simulink model "ModeStEnCtrl4s"  (R2018b)
settings: Solver=FixedStepDiscrete  StartTime=0.0  StopTime=10.0  FixedStep=0.01  RelTol=1e-3
undefined symbols (not defined in the file): EZE4sLStEnCtrl_Cal, EZE4sRStEnCtrl_Cal, EZQ4sLStEnCtrl_Cal, EZQ4sRStEnCtrl_Cal, FirstTrig, FwdLStEnCtrl_Cal, FwdRStEnCtrl_Cal, LgrstClsLStEnCtrl_Cal, LgrstClsRStEnCtrl_Cal, LgrstOpnLStEnCtrl_Cal, LgrstOpnRStEnCtrl_Cal, LyLStEnCtrl_Cal, LyRStEnCtrl_Cal, RecvL4sStEnCtrl_Cal, RecvR4sStEnCtrl_Cal, ResetCond, VIPL3582StEnCtrl_Cal, VIPL4sStEnCtrl_Cal, VIPR3582StEnCtrl_Cal, VIPR4sStEnCtrl_Cal, WelcomeBkwdStEnCtrl_Cal, WelcomeFwdStEnCtrl_Cal
libraries: simulink x20
settings Model: ModifiedHistory=2023.8.1 V2.0.0 CR421790 增加模式21-26  Creator=sn2xws  LastModifiedBy=sn55gm
settings DataIOCC: SaveFormat=StructureWithTime
settings OptimizationCC: DefaultParameterBehavior=Inlined  EnhancedBackFolding=on  PassReuseOutputArgsAs=Individual arguments  ZeroExternalMemoryAtStartup=off  ZeroInternalMemoryAtStartup=off  OptimizeBlockOrder=speed  DifferentSizesBufferReuse=on  OptimizationCustomize=off
settings DebuggingCC: ParameterTunabilityLossMsg=error
settings SFSimCC: MATLABDynamicMemAlloc=off
settings RTWCC: SystemTargetFile=autosar.tlc  GenCodeOnly=on  TemplateMakefile=ert_default_tmf  Description=AUTOSAR  GenerateReport=on  IncludeHyperlinkInReport=on  LaunchReport=on  GenerateTraceInfo=on  GenerateTraceReport=on  GenerateTraceReportSl=on  GenerateTraceReportSf=on  GenerateTraceReportEml=on  GenerateCodeMetricsReport=on
settings CodeAppCC: ForceParamTrailComments=on  IgnoreCustomStorageClasses=off  OperatorAnnotations=on  SimulinkDataObjDesc=on  SFDataObjDesc=on  InsertBlockDesc=on
settings STFCustomTargetCC: TargetLangStandard=C99 (ISO)  MultiwordLength=256  ParMdlRefBuildCompliant=on  CompOptLevelCompliant=on  IncludeMdlTerminateFcn=off  CombineOutputUpdateFcns=on  SuppressErrorStatus=on  ERTCustomFileBanners=on  SupportNonFinite=off  SupportComplex=off  SupportContinuousTime=off  SupportNonInlinedSFcns=off  RemoveResetFunc=on  MATLABClassNameForMDSCustomization=Simulink.SoftwareTarget.ERTCustomization  AutosarCompliant=on  UseToolchainInfoCompliant=on  LookupTableObjectStructAxisOrder=2,1,3,4,...  LUTObjectStructOrderEvenSpacing=Size,Table,Breakpoints  SystemTargetFile=autosar.tlc
settings ERTTargetCC: TargetLangStandard=C99 (ISO)  ConcurrentExecutionCompliant=off  IncludeMdlTerminateFcn=off  SuppressErrorStatus=on  SupportNonFinite=off  SupportComplex=off  ModelStepFunctionPrototypeControlCompliant=off  CPPClassGenCompliant=off  AutosarCompliant=on  LookupTableObjectStructAxisOrder=2,1,3,4,...  LUTObjectStructOrderEvenSpacing=Size,Table,Breakpoints  InlinedParameterPlacement=NonHierarchical  ERTCustomFileTemplate=example_file_process.tlc  ERTFilePackagingFormat=Compact

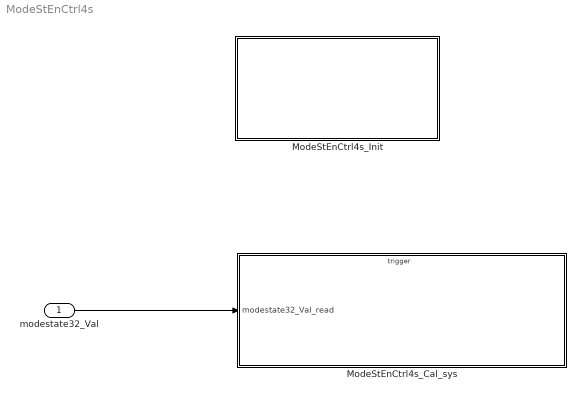
== system ModeStEnCtrl4s ==
  modestate32_Val : Inport  OutDataTypeStr=uint32  PortDimensions=1
  ModeStEnCtrl4s_Cal_sys : Subsystem
  ModeStEnCtrl4s_Init : Subsystem
  wires:
  modestate32_Val/1 -> ModeStEnCtrl4s_Cal_sys/1(modestate32_Val_read)

== system ModeStEnCtrl4s/ModeStEnCtrl4s_Cal_sys ==
  modestate32_Val_read : Inport
  function : TriggerPort  TriggerType=function-call  IsSimulinkFunction=on  FunctionName=ModeStEnCtrl4s_Cal  VariantControl=(inherit)
  Subsystem : Subsystem
  wires:
  modestate32_Val_read/1 -> Subsystem/1(modestate32_Val_read)

== system ModeStEnCtrl4s/ModeStEnCtrl4s_Init ==
  Event Listener : EventListener  EventName=reset

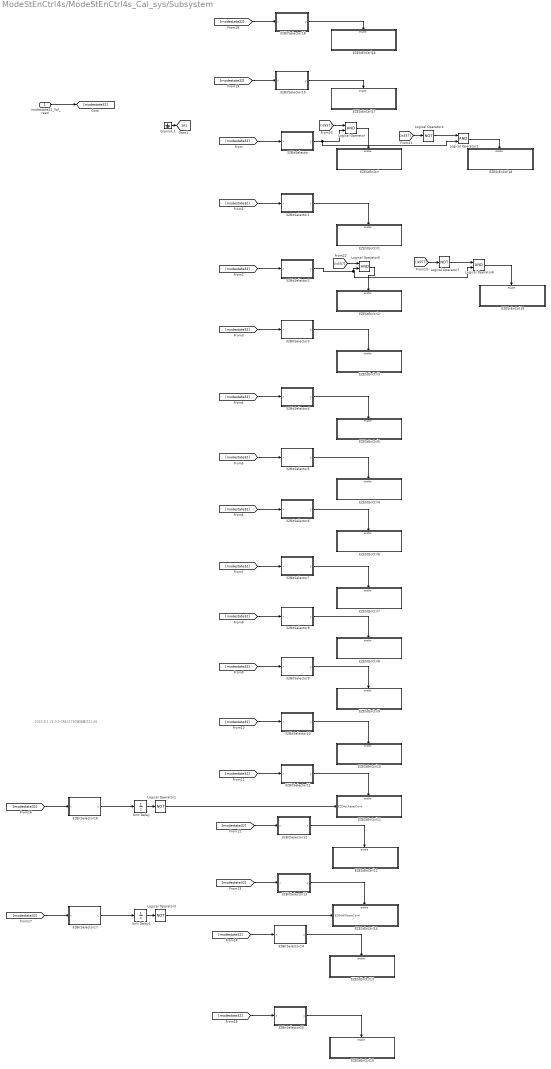
== system ModeStEnCtrl4s/ModeStEnCtrl4s_Cal_sys/Subsystem ==
  note: 2023.8.1 V2.0.0 CR421790 增加模式21-26
  modestate32_Val_read : Inport
  32BitSelector : Subsystem  mask(32 Bit Selector){BitNum=9}
      mask prompts: BitNum "Select Bit Number"
      mask help: Allows selection of a particular bit (0-31) out of a packed word up to 32 bits long. Output will be true if the bit number selected via the mask parameter is equal to one.
      mask TypeOptions BitNum: 0 | 1 | 2 | 3 | 4 | 5 | 6 | 7 | 8 | 9 | 10 | 11 | 12 | 13 | 14 | 15 | 16 | 17 | 18 | 19 | 20 | 21 | 22 | 23 | 24 | 25 | 26 | 27 | 28 | 29 | 30 | 31
      mask Display:
      | text(0.5, 0.8,'BIT','horizontalAlignment','center')
      | text(0.5, 0.5,'SELECTOR','horizontalAlignment','center')
      | text(0.5, 0.2,['-- Bit ',char(get_param(gcb,'BitNum')),' --'],'horizontalAlignment','center')
  32BitSelector1 : Subsystem  mask(32 Bit Selector){BitNum=10}
      mask prompts: BitNum "Select Bit Number"
      mask help: Allows selection of a particular bit (0-31) out of a packed word up to 32 bits long. Output will be true if the bit number selected via the mask parameter is equal to one.
      mask TypeOptions BitNum: 0 | 1 | 2 | 3 | 4 | 5 | 6 | 7 | 8 | 9 | 10 | 11 | 12 | 13 | 14 | 15 | 16 | 17 | 18 | 19 | 20 | 21 | 22 | 23 | 24 | 25 | 26 | 27 | 28 | 29 | 30 | 31
      mask Display:
      | text(0.5, 0.8,'BIT','horizontalAlignment','center')
      | text(0.5, 0.5,'SELECTOR','horizontalAlignment','center')
      | text(0.5, 0.2,['-- Bit ',char(get_param(gcb,'BitNum')),' --'],'horizontalAlignment','center')
  32BitSelector10 : Subsystem  mask(32 Bit Selector){BitNum=20}
      mask prompts: BitNum "Select Bit Number"
      mask help: Allows selection of a particular bit (0-31) out of a packed word up to 32 bits long. Output will be true if the bit number selected via the mask parameter is equal to one.
      mask TypeOptions BitNum: 0 | 1 | 2 | 3 | 4 | 5 | 6 | 7 | 8 | 9 | 10 | 11 | 12 | 13 | 14 | 15 | 16 | 17 | 18 | 19 | 20 | 21 | 22 | 23 | 24 | 25 | 26 | 27 | 28 | 29 | 30 | 31
      mask Display:
      | text(0.5, 0.8,'BIT','horizontalAlignment','center')
      | text(0.5, 0.5,'SELECTOR','horizontalAlignment','center')
      | text(0.5, 0.2,['-- Bit ',char(get_param(gcb,'BitNum')),' --'],'horizontalAlignment','center')
  32BitSelector11 : Subsystem  mask(32 Bit Selector){BitNum=21}
      mask prompts: BitNum "Select Bit Number"
      mask help: Allows selection of a particular bit (0-31) out of a packed word up to 32 bits long. Output will be true if the bit number selected via the mask parameter is equal to one.
      mask TypeOptions BitNum: 0 | 1 | 2 | 3 | 4 | 5 | 6 | 7 | 8 | 9 | 10 | 11 | 12 | 13 | 14 | 15 | 16 | 17 | 18 | 19 | 20 | 21 | 22 | 23 | 24 | 25 | 26 | 27 | 28 | 29 | 30 | 31
      mask Display:
      | text(0.5, 0.8,'BIT','horizontalAlignment','center')
      | text(0.5, 0.5,'SELECTOR','horizontalAlignment','center')
      | text(0.5, 0.2,['-- Bit ',char(get_param(gcb,'BitNum')),' --'],'horizontalAlignment','center')
  32BitSelector12 : Subsystem  mask(32 Bit Selector){BitNum=22}
      mask prompts: BitNum "Select Bit Number"
      mask help: Allows selection of a particular bit (0-31) out of a packed word up to 32 bits long. Output will be true if the bit number selected via the mask parameter is equal to one.
      mask TypeOptions BitNum: 0 | 1 | 2 | 3 | 4 | 5 | 6 | 7 | 8 | 9 | 10 | 11 | 12 | 13 | 14 | 15 | 16 | 17 | 18 | 19 | 20 | 21 | 22 | 23 | 24 | 25 | 26 | 27 | 28 | 29 | 30 | 31
      mask Display:
      | text(0.5, 0.8,'BIT','horizontalAlignment','center')
      | text(0.5, 0.5,'SELECTOR','horizontalAlignment','center')
      | text(0.5, 0.2,['-- Bit ',char(get_param(gcb,'BitNum')),' --'],'horizontalAlignment','center')
  32BitSelector13 : Subsystem  mask(32 Bit Selector){BitNum=23}
      mask prompts: BitNum "Select Bit Number"
      mask help: Allows selection of a particular bit (0-31) out of a packed word up to 32 bits long. Output will be true if the bit number selected via the mask parameter is equal to one.
      mask TypeOptions BitNum: 0 | 1 | 2 | 3 | 4 | 5 | 6 | 7 | 8 | 9 | 10 | 11 | 12 | 13 | 14 | 15 | 16 | 17 | 18 | 19 | 20 | 21 | 22 | 23 | 24 | 25 | 26 | 27 | 28 | 29 | 30 | 31
      mask Display:
      | text(0.5, 0.8,'BIT','horizontalAlignment','center')
      | text(0.5, 0.5,'SELECTOR','horizontalAlignment','center')
      | text(0.5, 0.2,['-- Bit ',char(get_param(gcb,'BitNum')),' --'],'horizontalAlignment','center')
  32BitSelector14 : Subsystem  mask(32 Bit Selector){BitNum=24}
      mask prompts: BitNum "Select Bit Number"
      mask help: Allows selection of a particular bit (0-31) out of a packed word up to 32 bits long. Output will be true if the bit number selected via the mask parameter is equal to one.
      mask TypeOptions BitNum: 0 | 1 | 2 | 3 | 4 | 5 | 6 | 7 | 8 | 9 | 10 | 11 | 12 | 13 | 14 | 15 | 16 | 17 | 18 | 19 | 20 | 21 | 22 | 23 | 24 | 25 | 26 | 27 | 28 | 29 | 30 | 31
      mask Display:
      | text(0.5, 0.8,'BIT','horizontalAlignment','center')
      | text(0.5, 0.5,'SELECTOR','horizontalAlignment','center')
      | text(0.5, 0.2,['-- Bit ',char(get_param(gcb,'BitNum')),' --'],'horizontalAlignment','center')
  32BitSelector15 : Subsystem  mask(32 Bit Selector){BitNum=25}
      mask prompts: BitNum "Select Bit Number"
      mask help: Allows selection of a particular bit (0-31) out of a packed word up to 32 bits long. Output will be true if the bit number selected via the mask parameter is equal to one.
      mask TypeOptions BitNum: 0 | 1 | 2 | 3 | 4 | 5 | 6 | 7 | 8 | 9 | 10 | 11 | 12 | 13 | 14 | 15 | 16 | 17 | 18 | 19 | 20 | 21 | 22 | 23 | 24 | 25 | 26 | 27 | 28 | 29 | 30 | 31
      mask Display:
      | text(0.5, 0.8,'BIT','horizontalAlignment','center')
      | text(0.5, 0.5,'SELECTOR','horizontalAlignment','center')
      | text(0.5, 0.2,['-- Bit ',char(get_param(gcb,'BitNum')),' --'],'horizontalAlignment','center')
  32BitSelector16 : Subsystem  mask(32 Bit Selector){BitNum=21}
      mask prompts: BitNum "Select Bit Number"
      mask help: Allows selection of a particular bit (0-31) out of a packed word up to 32 bits long. Output will be true if the bit number selected via the mask parameter is equal to one.
      mask TypeOptions BitNum: 0 | 1 | 2 | 3 | 4 | 5 | 6 | 7 | 8 | 9 | 10 | 11 | 12 | 13 | 14 | 15 | 16 | 17 | 18 | 19 | 20 | 21 | 22 | 23 | 24 | 25 | 26 | 27 | 28 | 29 | 30 | 31
      mask Display:
      | text(0.5, 0.8,'BIT','horizontalAlignment','center')
      | text(0.5, 0.5,'SELECTOR','horizontalAlignment','center')
      | text(0.5, 0.2,['-- Bit ',char(get_param(gcb,'BitNum')),' --'],'horizontalAlignment','center')
  32BitSelector17 : Subsystem  mask(32 Bit Selector){BitNum=23}
      mask prompts: BitNum "Select Bit Number"
      mask help: Allows selection of a particular bit (0-31) out of a packed word up to 32 bits long. Output will be true if the bit number selected via the mask parameter is equal to one.
      mask TypeOptions BitNum: 0 | 1 | 2 | 3 | 4 | 5 | 6 | 7 | 8 | 9 | 10 | 11 | 12 | 13 | 14 | 15 | 16 | 17 | 18 | 19 | 20 | 21 | 22 | 23 | 24 | 25 | 26 | 27 | 28 | 29 | 30 | 31
      mask Display:
      | text(0.5, 0.8,'BIT','horizontalAlignment','center')
      | text(0.5, 0.5,'SELECTOR','horizontalAlignment','center')
      | text(0.5, 0.2,['-- Bit ',char(get_param(gcb,'BitNum')),' --'],'horizontalAlignment','center')
  32BitSelector18 : Subsystem  mask(32 Bit Selector){BitNum=5}
      mask prompts: BitNum "Select Bit Number"
      mask help: Allows selection of a particular bit (0-31) out of a packed word up to 32 bits long. Output will be true if the bit number selected via the mask parameter is equal to one.
      mask TypeOptions BitNum: 0 | 1 | 2 | 3 | 4 | 5 | 6 | 7 | 8 | 9 | 10 | 11 | 12 | 13 | 14 | 15 | 16 | 17 | 18 | 19 | 20 | 21 | 22 | 23 | 24 | 25 | 26 | 27 | 28 | 29 | 30 | 31
      mask Display:
      | text(0.5, 0.8,'BIT','horizontalAlignment','center')
      | text(0.5, 0.5,'SELECTOR','horizontalAlignment','center')
      | text(0.5, 0.2,['-- Bit ',char(get_param(gcb,'BitNum')),' --'],'horizontalAlignment','center')
  32BitSelector19 : Subsystem  mask(32 Bit Selector){BitNum=6}
      mask prompts: BitNum "Select Bit Number"
      mask help: Allows selection of a particular bit (0-31) out of a packed word up to 32 bits long. Output will be true if the bit number selected via the mask parameter is equal to one.
      mask TypeOptions BitNum: 0 | 1 | 2 | 3 | 4 | 5 | 6 | 7 | 8 | 9 | 10 | 11 | 12 | 13 | 14 | 15 | 16 | 17 | 18 | 19 | 20 | 21 | 22 | 23 | 24 | 25 | 26 | 27 | 28 | 29 | 30 | 31
      mask Display:
      | text(0.5, 0.8,'BIT','horizontalAlignment','center')
      | text(0.5, 0.5,'SELECTOR','horizontalAlignment','center')
      | text(0.5, 0.2,['-- Bit ',char(get_param(gcb,'BitNum')),' --'],'horizontalAlignment','center')
  32BitSelector2 : Subsystem  mask(32 Bit Selector){BitNum=11}
      mask prompts: BitNum "Select Bit Number"
      mask help: Allows selection of a particular bit (0-31) out of a packed word up to 32 bits long. Output will be true if the bit number selected via the mask parameter is equal to one.
      mask TypeOptions BitNum: 0 | 1 | 2 | 3 | 4 | 5 | 6 | 7 | 8 | 9 | 10 | 11 | 12 | 13 | 14 | 15 | 16 | 17 | 18 | 19 | 20 | 21 | 22 | 23 | 24 | 25 | 26 | 27 | 28 | 29 | 30 | 31
      mask Display:
      | text(0.5, 0.8,'BIT','horizontalAlignment','center')
      | text(0.5, 0.5,'SELECTOR','horizontalAlignment','center')
      | text(0.5, 0.2,['-- Bit ',char(get_param(gcb,'BitNum')),' --'],'horizontalAlignment','center')
  32BitSelector3 : Subsystem  mask(32 Bit Selector){BitNum=12}
      mask prompts: BitNum "Select Bit Number"
      mask help: Allows selection of a particular bit (0-31) out of a packed word up to 32 bits long. Output will be true if the bit number selected via the mask parameter is equal to one.
      mask TypeOptions BitNum: 0 | 1 | 2 | 3 | 4 | 5 | 6 | 7 | 8 | 9 | 10 | 11 | 12 | 13 | 14 | 15 | 16 | 17 | 18 | 19 | 20 | 21 | 22 | 23 | 24 | 25 | 26 | 27 | 28 | 29 | 30 | 31
      mask Display:
      | text(0.5, 0.8,'BIT','horizontalAlignment','center')
      | text(0.5, 0.5,'SELECTOR','horizontalAlignment','center')
      | text(0.5, 0.2,['-- Bit ',char(get_param(gcb,'BitNum')),' --'],'horizontalAlignment','center')
  32BitSelector4 : Subsystem  mask(32 Bit Selector){BitNum=13}
      mask prompts: BitNum "Select Bit Number"
      mask help: Allows selection of a particular bit (0-31) out of a packed word up to 32 bits long. Output will be true if the bit number selected via the mask parameter is equal to one.
      mask TypeOptions BitNum: 0 | 1 | 2 | 3 | 4 | 5 | 6 | 7 | 8 | 9 | 10 | 11 | 12 | 13 | 14 | 15 | 16 | 17 | 18 | 19 | 20 | 21 | 22 | 23 | 24 | 25 | 26 | 27 | 28 | 29 | 30 | 31
      mask Display:
      | text(0.5, 0.8,'BIT','horizontalAlignment','center')
      | text(0.5, 0.5,'SELECTOR','horizontalAlignment','center')
      | text(0.5, 0.2,['-- Bit ',char(get_param(gcb,'BitNum')),' --'],'horizontalAlignment','center')
  32BitSelector5 : Subsystem  mask(32 Bit Selector){BitNum=14}
      mask prompts: BitNum "Select Bit Number"
      mask help: Allows selection of a particular bit (0-31) out of a packed word up to 32 bits long. Output will be true if the bit number selected via the mask parameter is equal to one.
      mask TypeOptions BitNum: 0 | 1 | 2 | 3 | 4 | 5 | 6 | 7 | 8 | 9 | 10 | 11 | 12 | 13 | 14 | 15 | 16 | 17 | 18 | 19 | 20 | 21 | 22 | 23 | 24 | 25 | 26 | 27 | 28 | 29 | 30 | 31
      mask Display:
      | text(0.5, 0.8,'BIT','horizontalAlignment','center')
      | text(0.5, 0.5,'SELECTOR','horizontalAlignment','center')
      | text(0.5, 0.2,['-- Bit ',char(get_param(gcb,'BitNum')),' --'],'horizontalAlignment','center')
  32BitSelector6 : Subsystem  mask(32 Bit Selector){BitNum=15}
      mask prompts: BitNum "Select Bit Number"
      mask help: Allows selection of a particular bit (0-31) out of a packed word up to 32 bits long. Output will be true if the bit number selected via the mask parameter is equal to one.
      mask TypeOptions BitNum: 0 | 1 | 2 | 3 | 4 | 5 | 6 | 7 | 8 | 9 | 10 | 11 | 12 | 13 | 14 | 15 | 16 | 17 | 18 | 19 | 20 | 21 | 22 | 23 | 24 | 25 | 26 | 27 | 28 | 29 | 30 | 31
      mask Display:
      | text(0.5, 0.8,'BIT','horizontalAlignment','center')
      | text(0.5, 0.5,'SELECTOR','horizontalAlignment','center')
      | text(0.5, 0.2,['-- Bit ',char(get_param(gcb,'BitNum')),' --'],'horizontalAlignment','center')
  32BitSelector7 : Subsystem  mask(32 Bit Selector){BitNum=16}
      mask prompts: BitNum "Select Bit Number"
      mask help: Allows selection of a particular bit (0-31) out of a packed word up to 32 bits long. Output will be true if the bit number selected via the mask parameter is equal to one.
      mask TypeOptions BitNum: 0 | 1 | 2 | 3 | 4 | 5 | 6 | 7 | 8 | 9 | 10 | 11 | 12 | 13 | 14 | 15 | 16 | 17 | 18 | 19 | 20 | 21 | 22 | 23 | 24 | 25 | 26 | 27 | 28 | 29 | 30 | 31
      mask Display:
      | text(0.5, 0.8,'BIT','horizontalAlignment','center')
      | text(0.5, 0.5,'SELECTOR','horizontalAlignment','center')
      | text(0.5, 0.2,['-- Bit ',char(get_param(gcb,'BitNum')),' --'],'horizontalAlignment','center')
  32BitSelector8 : Subsystem  mask(32 Bit Selector){BitNum=17}
      mask prompts: BitNum "Select Bit Number"
      mask help: Allows selection of a particular bit (0-31) out of a packed word up to 32 bits long. Output will be true if the bit number selected via the mask parameter is equal to one.
      mask TypeOptions BitNum: 0 | 1 | 2 | 3 | 4 | 5 | 6 | 7 | 8 | 9 | 10 | 11 | 12 | 13 | 14 | 15 | 16 | 17 | 18 | 19 | 20 | 21 | 22 | 23 | 24 | 25 | 26 | 27 | 28 | 29 | 30 | 31
      mask Display:
      | text(0.5, 0.8,'BIT','horizontalAlignment','center')
      | text(0.5, 0.5,'SELECTOR','horizontalAlignment','center')
      | text(0.5, 0.2,['-- Bit ',char(get_param(gcb,'BitNum')),' --'],'horizontalAlignment','center')
  32BitSelector9 : Subsystem  mask(32 Bit Selector){BitNum=18}
      mask prompts: BitNum "Select Bit Number"
      mask help: Allows selection of a particular bit (0-31) out of a packed word up to 32 bits long. Output will be true if the bit number selected via the mask parameter is equal to one.
      mask TypeOptions BitNum: 0 | 1 | 2 | 3 | 4 | 5 | 6 | 7 | 8 | 9 | 10 | 11 | 12 | 13 | 14 | 15 | 16 | 17 | 18 | 19 | 20 | 21 | 22 | 23 | 24 | 25 | 26 | 27 | 28 | 29 | 30 | 31
      mask Display:
      | text(0.5, 0.8,'BIT','horizontalAlignment','center')
      | text(0.5, 0.5,'SELECTOR','horizontalAlignment','center')
      | text(0.5, 0.2,['-- Bit ',char(get_param(gcb,'BitNum')),' --'],'horizontalAlignment','center')
  EZEStEnCtrl : Subsystem  TreatAsAtomicUnit=on
  EZEStEnCtrl1 : Subsystem  TreatAsAtomicUnit=on
  EZEStEnCtrl10 : Subsystem  TreatAsAtomicUnit=on
  EZEStEnCtrl11 : Subsystem  TreatAsAtomicUnit=on
  EZEStEnCtrl12 : Subsystem  TreatAsAtomicUnit=on
  EZEStEnCtrl13 : Subsystem  TreatAsAtomicUnit=on
  EZEStEnCtrl14 : Subsystem  TreatAsAtomicUnit=on
  EZEStEnCtrl15 : Subsystem  TreatAsAtomicUnit=on
  EZEStEnCtrl16 : Subsystem  TreatAsAtomicUnit=on
  EZEStEnCtrl17 : Subsystem  TreatAsAtomicUnit=on
  EZEStEnCtrl18 : Subsystem  TreatAsAtomicUnit=on
  EZEStEnCtrl19 : Subsystem  TreatAsAtomicUnit=on
  EZEStEnCtrl2 : Subsystem  TreatAsAtomicUnit=on
  EZEStEnCtrl3 : Subsystem  TreatAsAtomicUnit=on
  EZEStEnCtrl4 : Subsystem  TreatAsAtomicUnit=on
  EZEStEnCtrl5 : Subsystem  TreatAsAtomicUnit=on
  EZEStEnCtrl6 : Subsystem  TreatAsAtomicUnit=on
  EZEStEnCtrl7 : Subsystem  TreatAsAtomicUnit=on
  EZEStEnCtrl8 : Subsystem  TreatAsAtomicUnit=on
  EZEStEnCtrl9 : Subsystem  TreatAsAtomicUnit=on
  Ground_1 : Ground
  Logical Operator{,2,5..6} (4 alike) : Logic  AllPortsSameDT=off  OutDataTypeStr=boolean
  Logical Operator{1,3..4,7} (4 alike) : Logic  Operator=NOT  AllPortsSameDT=off  OutDataTypeStr=boolean
  Unit Delay : UnitDelay  SampleTime=-1
  Unit Delay1 : UnitDelay  SampleTime=-1
  wires:
  [modestate32] -> 32BitSelector/1(x)
  modestate32_Val_read/1 -> [modestate32]
  [modestate32] -> 32BitSelector1/1(x)
  32BitSelector1/1(y) -> EZEStEnCtrl1/Enable
  [modestate32] -> 32BitSelector2/1(x)
  [modestate32] -> 32BitSelector3/1(x)
  32BitSelector3/1(y) -> EZEStEnCtrl3/Enable
  32BitSelector4/1(y) -> EZEStEnCtrl5/Enable
  [modestate32] -> 32BitSelector4/1(x)
  [modestate32] -> 32BitSelector5/1(x)
  32BitSelector5/1(y) -> EZEStEnCtrl4/Enable
  32BitSelector6/1(y) -> EZEStEnCtrl6/Enable
  [modestate32] -> 32BitSelector6/1(x)
  [modestate32] -> 32BitSelector7/1(x)
  32BitSelector7/1(y) -> EZEStEnCtrl7/Enable
  32BitSelector8/1(y) -> EZEStEnCtrl8/Enable
  [modestate32] -> 32BitSelector8/1(x)
  [modestate32] -> 32BitSelector9/1(x)
  32BitSelector9/1(y) -> EZEStEnCtrl9/Enable
  32BitSelector10/1(y) -> EZEStEnCtrl10/Enable
  [modestate32] -> 32BitSelector10/1(x)
  [modestate32] -> 32BitSelector11/1(x)
  32BitSelector11/1(y) -> EZEStEnCtrl11/Enable
  32BitSelector12/1(y) -> EZEStEnCtrl12/Enable
  [modestate32] -> 32BitSelector12/1(x)
  [modestate32] -> 32BitSelector13/1(x)
  32BitSelector13/1(y) -> EZEStEnCtrl14/Enable
  32BitSelector14/1(y) -> EZEStEnCtrl13/Enable
  [modestate32] -> 32BitSelector14/1(x)
  [modestate32] -> 32BitSelector15/1(x)
  32BitSelector15/1(y) -> EZEStEnCtrl15/Enable
  Logical Operator1/1 -> EZEStEnCtrl11/1(EZQ4sLResetCond)
  [modestate32] -> 32BitSelector16/1(x)
  32BitSelector16/1(y) -> Unit Delay/1
  Unit Delay/1 -> Logical Operator1/1
  Unit Delay1/1 -> Logical Operator3/1
  32BitSelector17/1(y) -> Unit Delay1/1
  [modestate32] -> 32BitSelector17/1(x)
  Logical Operator3/1 -> EZEStEnCtrl14/1(EZQ4sRResetCond)
  32BitSelector18/1(y) -> EZEStEnCtrl16/Enable
  [modestate32] -> 32BitSelector18/1(x)
  32BitSelector19/1(y) -> EZEStEnCtrl17/Enable
  [modestate32] -> 32BitSelector19/1(x)
  [is557] -> Logical Operator/1
  32BitSelector/1(y) -> Logical Operator2/2, Logical Operator/2
  Logical Operator/1 -> EZEStEnCtrl/Enable
  [is557] -> Logical Operator4/1
  Logical Operator4/1 -> Logical Operator2/1
  Logical Operator2/1 -> EZEStEnCtrl18/Enable
  [is557] -> Logical Operator5/1
  Logical Operator5/1 -> EZEStEnCtrl2/Enable
  32BitSelector2/1(y) -> Logical Operator6/2, Logical Operator5/2
  Logical Operator7/1 -> Logical Operator6/1
  [is557] -> Logical Operator7/1
  Logical Operator6/1 -> EZEStEnCtrl19/Enable
  Ground_1/1 -> [A]

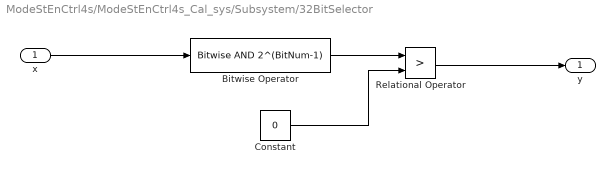
== system ModeStEnCtrl4s/ModeStEnCtrl4s_Cal_sys/Subsystem/32BitSelector ==
  x : Inport
  Bitwise Operator : simulink/Logic and Bit Operations/Bitwise Operator  logicop=AND  UseBitMask=on  BitMask=2^(BitNum-1)  BitMaskRealWorld=Stored Integer
  Constant : Constant  Value=0  OutDataTypeStr=uint32
  Relational Operator : RelationalOperator  Operator=>  OutDataTypeStr=boolean  RndMeth=Simplest
  y : Outport
  wires:
  Relational Operator/1 -> y/1
  Constant/1 -> Relational Operator/2
  x/1 -> Bitwise Operator/1
  Bitwise Operator/1 -> Relational Operator/1

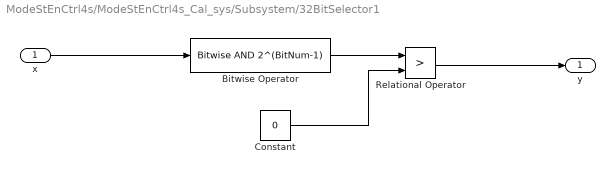
== system ModeStEnCtrl4s/ModeStEnCtrl4s_Cal_sys/Subsystem/32BitSelector1 ==
  x : Inport
  Bitwise Operator : simulink/Logic and Bit Operations/Bitwise Operator  logicop=AND  UseBitMask=on  BitMask=2^(BitNum-1)  BitMaskRealWorld=Stored Integer
  Constant : Constant  Value=0  OutDataTypeStr=uint32
  Relational Operator : RelationalOperator  Operator=>  OutDataTypeStr=boolean  RndMeth=Simplest
  y : Outport
  wires:
  Bitwise Operator/1 -> Relational Operator/1
  x/1 -> Bitwise Operator/1
  Constant/1 -> Relational Operator/2
  Relational Operator/1 -> y/1

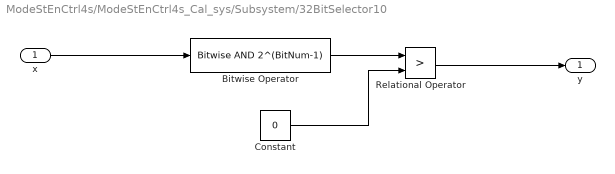
== system ModeStEnCtrl4s/ModeStEnCtrl4s_Cal_sys/Subsystem/32BitSelector10 ==
  x : Inport
  Bitwise Operator : simulink/Logic and Bit Operations/Bitwise Operator  logicop=AND  UseBitMask=on  BitMask=2^(BitNum-1)  BitMaskRealWorld=Stored Integer
  Constant : Constant  Value=0  OutDataTypeStr=uint32
  Relational Operator : RelationalOperator  Operator=>  OutDataTypeStr=boolean  RndMeth=Simplest
  y : Outport
  wires:
  Relational Operator/1 -> y/1
  Constant/1 -> Relational Operator/2
  x/1 -> Bitwise Operator/1
  Bitwise Operator/1 -> Relational Operator/1

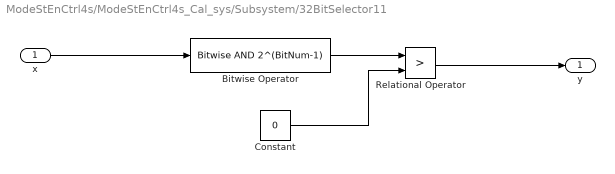
== system ModeStEnCtrl4s/ModeStEnCtrl4s_Cal_sys/Subsystem/32BitSelector11 ==
  x : Inport
  Bitwise Operator : simulink/Logic and Bit Operations/Bitwise Operator  logicop=AND  UseBitMask=on  BitMask=2^(BitNum-1)  BitMaskRealWorld=Stored Integer
  Constant : Constant  Value=0  OutDataTypeStr=uint32
  Relational Operator : RelationalOperator  Operator=>  OutDataTypeStr=boolean  RndMeth=Simplest
  y : Outport
  wires:
  Bitwise Operator/1 -> Relational Operator/1
  x/1 -> Bitwise Operator/1
  Constant/1 -> Relational Operator/2
  Relational Operator/1 -> y/1

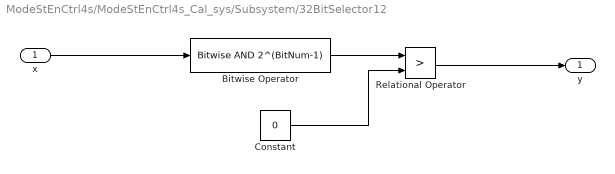
== system ModeStEnCtrl4s/ModeStEnCtrl4s_Cal_sys/Subsystem/32BitSelector12 ==
  x : Inport
  Bitwise Operator : simulink/Logic and Bit Operations/Bitwise Operator  logicop=AND  UseBitMask=on  BitMask=2^(BitNum-1)  BitMaskRealWorld=Stored Integer
  Constant : Constant  Value=0  OutDataTypeStr=uint32
  Relational Operator : RelationalOperator  Operator=>  OutDataTypeStr=boolean  RndMeth=Simplest
  y : Outport
  wires:
  Relational Operator/1 -> y/1
  Constant/1 -> Relational Operator/2
  x/1 -> Bitwise Operator/1
  Bitwise Operator/1 -> Relational Operator/1

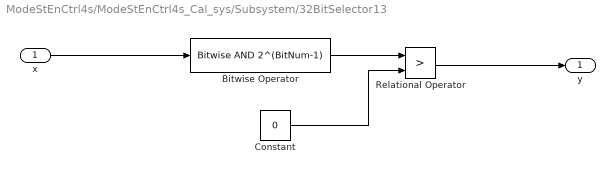
== system ModeStEnCtrl4s/ModeStEnCtrl4s_Cal_sys/Subsystem/32BitSelector13 ==
  x : Inport
  Bitwise Operator : simulink/Logic and Bit Operations/Bitwise Operator  logicop=AND  UseBitMask=on  BitMask=2^(BitNum-1)  BitMaskRealWorld=Stored Integer
  Constant : Constant  Value=0  OutDataTypeStr=uint32
  Relational Operator : RelationalOperator  Operator=>  OutDataTypeStr=boolean  RndMeth=Simplest
  y : Outport
  wires:
  Bitwise Operator/1 -> Relational Operator/1
  x/1 -> Bitwise Operator/1
  Constant/1 -> Relational Operator/2
  Relational Operator/1 -> y/1

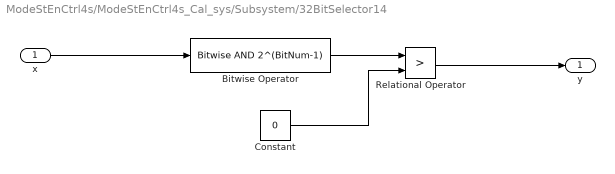
== system ModeStEnCtrl4s/ModeStEnCtrl4s_Cal_sys/Subsystem/32BitSelector14 ==
  x : Inport
  Bitwise Operator : simulink/Logic and Bit Operations/Bitwise Operator  logicop=AND  UseBitMask=on  BitMask=2^(BitNum-1)  BitMaskRealWorld=Stored Integer
  Constant : Constant  Value=0  OutDataTypeStr=uint32
  Relational Operator : RelationalOperator  Operator=>  OutDataTypeStr=boolean  RndMeth=Simplest
  y : Outport
  wires:
  Relational Operator/1 -> y/1
  Constant/1 -> Relational Operator/2
  x/1 -> Bitwise Operator/1
  Bitwise Operator/1 -> Relational Operator/1

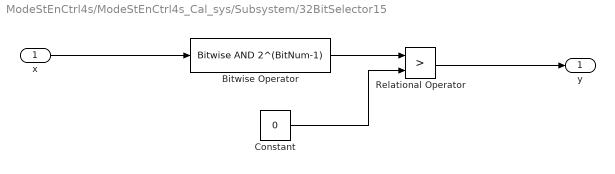
== system ModeStEnCtrl4s/ModeStEnCtrl4s_Cal_sys/Subsystem/32BitSelector15 ==
  x : Inport
  Bitwise Operator : simulink/Logic and Bit Operations/Bitwise Operator  logicop=AND  UseBitMask=on  BitMask=2^(BitNum-1)  BitMaskRealWorld=Stored Integer
  Constant : Constant  Value=0  OutDataTypeStr=uint32
  Relational Operator : RelationalOperator  Operator=>  OutDataTypeStr=boolean  RndMeth=Simplest
  y : Outport
  wires:
  Bitwise Operator/1 -> Relational Operator/1
  x/1 -> Bitwise Operator/1
  Constant/1 -> Relational Operator/2
  Relational Operator/1 -> y/1

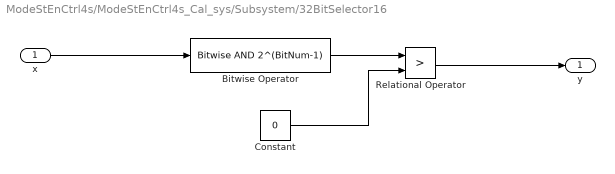
== system ModeStEnCtrl4s/ModeStEnCtrl4s_Cal_sys/Subsystem/32BitSelector16 ==
  x : Inport
  Bitwise Operator : simulink/Logic and Bit Operations/Bitwise Operator  logicop=AND  UseBitMask=on  BitMask=2^(BitNum-1)  BitMaskRealWorld=Stored Integer
  Constant : Constant  Value=0  OutDataTypeStr=uint32
  Relational Operator : RelationalOperator  Operator=>  OutDataTypeStr=boolean  RndMeth=Simplest
  y : Outport
  wires:
  Relational Operator/1 -> y/1
  Constant/1 -> Relational Operator/2
  x/1 -> Bitwise Operator/1
  Bitwise Operator/1 -> Relational Operator/1

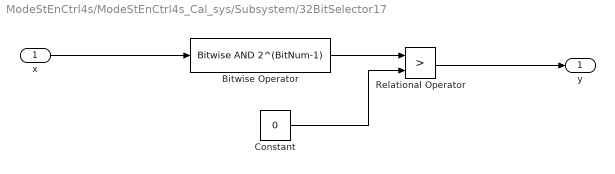
== system ModeStEnCtrl4s/ModeStEnCtrl4s_Cal_sys/Subsystem/32BitSelector17 ==
  x : Inport
  Bitwise Operator : simulink/Logic and Bit Operations/Bitwise Operator  logicop=AND  UseBitMask=on  BitMask=2^(BitNum-1)  BitMaskRealWorld=Stored Integer
  Constant : Constant  Value=0  OutDataTypeStr=uint32
  Relational Operator : RelationalOperator  Operator=>  OutDataTypeStr=boolean  RndMeth=Simplest
  y : Outport
  wires:
  Bitwise Operator/1 -> Relational Operator/1
  x/1 -> Bitwise Operator/1
  Constant/1 -> Relational Operator/2
  Relational Operator/1 -> y/1

== system ModeStEnCtrl4s/ModeStEnCtrl4s_Cal_sys/Subsystem/32BitSelector18 ==
  x : Inport
  Bitwise Operator : simulink/Logic and Bit Operations/Bitwise Operator  logicop=AND  UseBitMask=on  BitMask=2^(BitNum-1)  BitMaskRealWorld=Stored Integer
  Constant : Constant  Value=0  OutDataTypeStr=uint32
  Relational Operator : RelationalOperator  Operator=>  OutDataTypeStr=boolean  RndMeth=Simplest
  y : Outport
  wires:
  Relational Operator/1 -> y/1
  Constant/1 -> Relational Operator/2
  x/1 -> Bitwise Operator/1
  Bitwise Operator/1 -> Relational Operator/1

== system ModeStEnCtrl4s/ModeStEnCtrl4s_Cal_sys/Subsystem/32BitSelector19 ==
  x : Inport
  Bitwise Operator : simulink/Logic and Bit Operations/Bitwise Operator  logicop=AND  UseBitMask=on  BitMask=2^(BitNum-1)  BitMaskRealWorld=Stored Integer
  Constant : Constant  Value=0  OutDataTypeStr=uint32
  Relational Operator : RelationalOperator  Operator=>  OutDataTypeStr=boolean  RndMeth=Simplest
  y : Outport
  wires:
  Relational Operator/1 -> y/1
  Constant/1 -> Relational Operator/2
  x/1 -> Bitwise Operator/1
  Bitwise Operator/1 -> Relational Operator/1

== system ModeStEnCtrl4s/ModeStEnCtrl4s_Cal_sys/Subsystem/32BitSelector2 ==
  x : Inport
  Bitwise Operator : simulink/Logic and Bit Operations/Bitwise Operator  logicop=AND  UseBitMask=on  BitMask=2^(BitNum-1)  BitMaskRealWorld=Stored Integer
  Constant : Constant  Value=0  OutDataTypeStr=uint32
  Relational Operator : RelationalOperator  Operator=>  OutDataTypeStr=boolean  RndMeth=Simplest
  y : Outport
  wires:
  Relational Operator/1 -> y/1
  Constant/1 -> Relational Operator/2
  x/1 -> Bitwise Operator/1
  Bitwise Operator/1 -> Relational Operator/1

== system ModeStEnCtrl4s/ModeStEnCtrl4s_Cal_sys/Subsystem/32BitSelector3 ==
  x : Inport
  Bitwise Operator : simulink/Logic and Bit Operations/Bitwise Operator  logicop=AND  UseBitMask=on  BitMask=2^(BitNum-1)  BitMaskRealWorld=Stored Integer
  Constant : Constant  Value=0  OutDataTypeStr=uint32
  Relational Operator : RelationalOperator  Operator=>  OutDataTypeStr=boolean  RndMeth=Simplest
  y : Outport
  wires:
  Bitwise Operator/1 -> Relational Operator/1
  x/1 -> Bitwise Operator/1
  Constant/1 -> Relational Operator/2
  Relational Operator/1 -> y/1

== system ModeStEnCtrl4s/ModeStEnCtrl4s_Cal_sys/Subsystem/32BitSelector4 ==
  x : Inport
  Bitwise Operator : simulink/Logic and Bit Operations/Bitwise Operator  logicop=AND  UseBitMask=on  BitMask=2^(BitNum-1)  BitMaskRealWorld=Stored Integer
  Constant : Constant  Value=0  OutDataTypeStr=uint32
  Relational Operator : RelationalOperator  Operator=>  OutDataTypeStr=boolean  RndMeth=Simplest
  y : Outport
  wires:
  Relational Operator/1 -> y/1
  Constant/1 -> Relational Operator/2
  x/1 -> Bitwise Operator/1
  Bitwise Operator/1 -> Relational Operator/1

== system ModeStEnCtrl4s/ModeStEnCtrl4s_Cal_sys/Subsystem/32BitSelector5 ==
  x : Inport
  Bitwise Operator : simulink/Logic and Bit Operations/Bitwise Operator  logicop=AND  UseBitMask=on  BitMask=2^(BitNum-1)  BitMaskRealWorld=Stored Integer
  Constant : Constant  Value=0  OutDataTypeStr=uint32
  Relational Operator : RelationalOperator  Operator=>  OutDataTypeStr=boolean  RndMeth=Simplest
  y : Outport
  wires:
  Bitwise Operator/1 -> Relational Operator/1
  x/1 -> Bitwise Operator/1
  Constant/1 -> Relational Operator/2
  Relational Operator/1 -> y/1

== system ModeStEnCtrl4s/ModeStEnCtrl4s_Cal_sys/Subsystem/32BitSelector6 ==
  x : Inport
  Bitwise Operator : simulink/Logic and Bit Operations/Bitwise Operator  logicop=AND  UseBitMask=on  BitMask=2^(BitNum-1)  BitMaskRealWorld=Stored Integer
  Constant : Constant  Value=0  OutDataTypeStr=uint32
  Relational Operator : RelationalOperator  Operator=>  OutDataTypeStr=boolean  RndMeth=Simplest
  y : Outport
  wires:
  Relational Operator/1 -> y/1
  Constant/1 -> Relational Operator/2
  x/1 -> Bitwise Operator/1
  Bitwise Operator/1 -> Relational Operator/1

== system ModeStEnCtrl4s/ModeStEnCtrl4s_Cal_sys/Subsystem/32BitSelector7 ==
  x : Inport
  Bitwise Operator : simulink/Logic and Bit Operations/Bitwise Operator  logicop=AND  UseBitMask=on  BitMask=2^(BitNum-1)  BitMaskRealWorld=Stored Integer
  Constant : Constant  Value=0  OutDataTypeStr=uint32
  Relational Operator : RelationalOperator  Operator=>  OutDataTypeStr=boolean  RndMeth=Simplest
  y : Outport
  wires:
  Bitwise Operator/1 -> Relational Operator/1
  x/1 -> Bitwise Operator/1
  Constant/1 -> Relational Operator/2
  Relational Operator/1 -> y/1

== system ModeStEnCtrl4s/ModeStEnCtrl4s_Cal_sys/Subsystem/32BitSelector8 ==
  x : Inport
  Bitwise Operator : simulink/Logic and Bit Operations/Bitwise Operator  logicop=AND  UseBitMask=on  BitMask=2^(BitNum-1)  BitMaskRealWorld=Stored Integer
  Constant : Constant  Value=0  OutDataTypeStr=uint32
  Relational Operator : RelationalOperator  Operator=>  OutDataTypeStr=boolean  RndMeth=Simplest
  y : Outport
  wires:
  Relational Operator/1 -> y/1
  Constant/1 -> Relational Operator/2
  x/1 -> Bitwise Operator/1
  Bitwise Operator/1 -> Relational Operator/1

== system ModeStEnCtrl4s/ModeStEnCtrl4s_Cal_sys/Subsystem/32BitSelector9 ==
  x : Inport
  Bitwise Operator : simulink/Logic and Bit Operations/Bitwise Operator  logicop=AND  UseBitMask=on  BitMask=2^(BitNum-1)  BitMaskRealWorld=Stored Integer
  Constant : Constant  Value=0  OutDataTypeStr=uint32
  Relational Operator : RelationalOperator  Operator=>  OutDataTypeStr=boolean  RndMeth=Simplest
  y : Outport
  wires:
  Bitwise Operator/1 -> Relational Operator/1
  x/1 -> Bitwise Operator/1
  Constant/1 -> Relational Operator/2
  Relational Operator/1 -> y/1

== system ModeStEnCtrl4s/ModeStEnCtrl4s_Cal_sys/Subsystem/EZEStEnCtrl ==
  note: Delete block
  Enable : EnablePort
  VIPL4sStEnCtrl_Cal : FunctionCaller  FunctionPrototype=VIPL4sStEnCtrl_Cal()

== system ModeStEnCtrl4s/ModeStEnCtrl4s_Cal_sys/Subsystem/EZEStEnCtrl1 ==
  note: Delete block
  Enable : EnablePort
  RecvL4sStEnCtrl_Cal : FunctionCaller  FunctionPrototype=RecvL4sStEnCtrl_Cal()

== system ModeStEnCtrl4s/ModeStEnCtrl4s_Cal_sys/Subsystem/EZEStEnCtrl10 ==
  note: Delete block
  Enable : EnablePort
  EZE4sLStEnCtrl_Cal : FunctionCaller  FunctionPrototype=EZE4sLStEnCtrl_Cal()

== system ModeStEnCtrl4s/ModeStEnCtrl4s_Cal_sys/Subsystem/EZEStEnCtrl11 ==
  note: Delete block
  EZQ4sLResetCond : Inport
  Enable : EnablePort
  EZQ4sLStEnCtrl_Cal : FunctionCaller  FunctionPrototype=EZQ4sLStEnCtrl_Cal(ResetCond)  InputArgumentSpecifications=boolean(true)
  wires:
  EZQ4sLResetCond/1 -> EZQ4sLStEnCtrl_Cal/1

== system ModeStEnCtrl4s/ModeStEnCtrl4s_Cal_sys/Subsystem/EZEStEnCtrl12 ==
  note: Delete block
  Enable : EnablePort
  EZE4sRStEnCtrl_Cal : FunctionCaller  FunctionPrototype=EZE4sRStEnCtrl_Cal()

== system ModeStEnCtrl4s/ModeStEnCtrl4s_Cal_sys/Subsystem/EZEStEnCtrl13 ==
  note: Delete block
  Enable : EnablePort
  WelcomeBkwdStEnCtrl_Cal : FunctionCaller  FunctionPrototype=WelcomeBkwdStEnCtrl_Cal()

== system ModeStEnCtrl4s/ModeStEnCtrl4s_Cal_sys/Subsystem/EZEStEnCtrl14 ==
  note: Delete block
  EZQ4sRResetCond : Inport
  Enable : EnablePort
  EZQ4sRStEnCtrl_Cal : FunctionCaller  FunctionPrototype=EZQ4sRStEnCtrl_Cal(ResetCond)  InputArgumentSpecifications=boolean(true)
  wires:
  EZQ4sRResetCond/1 -> EZQ4sRStEnCtrl_Cal/1

== system ModeStEnCtrl4s/ModeStEnCtrl4s_Cal_sys/Subsystem/EZEStEnCtrl15 ==
  note: Delete block
  Enable : EnablePort
  WelcomeFwdStEnCtrl_Cal : FunctionCaller  FunctionPrototype=WelcomeFwdStEnCtrl_Cal()

== system ModeStEnCtrl4s/ModeStEnCtrl4s_Cal_sys/Subsystem/EZEStEnCtrl16 ==
  Enable : EnablePort
  FwdLStEnCtrl_Cal : FunctionCaller  FunctionPrototype=FwdLStEnCtrl_Cal()

== system ModeStEnCtrl4s/ModeStEnCtrl4s_Cal_sys/Subsystem/EZEStEnCtrl17 ==
  Enable : EnablePort
  FwdRStEnCtrl_Cal : FunctionCaller  FunctionPrototype=FwdRStEnCtrl_Cal()

== system ModeStEnCtrl4s/ModeStEnCtrl4s_Cal_sys/Subsystem/EZEStEnCtrl18 ==
  note: Delete block
  Enable : EnablePort
  VIPL3582StEnCtrl_Cal : FunctionCaller  FunctionPrototype=VIPL3582StEnCtrl_Cal()

== system ModeStEnCtrl4s/ModeStEnCtrl4s_Cal_sys/Subsystem/EZEStEnCtrl19 ==
  note: Delete block
  Enable : EnablePort
  Constant : Constant  Value=0  OutDataTypeStr=boolean
  Unit Delay : UnitDelay  InitialCondition=1  SampleTime=-1
  VIPR3582StEnCtrl_Cal : FunctionCaller  FunctionPrototype=VIPR3582StEnCtrl_Cal(FirstTrig)  InputArgumentSpecifications=boolean(true)
  wires:
  Constant/1 -> Unit Delay/1
  Unit Delay/1 -> VIPR3582StEnCtrl_Cal/1

== system ModeStEnCtrl4s/ModeStEnCtrl4s_Cal_sys/Subsystem/EZEStEnCtrl2 ==
  note: Delete block
  Enable : EnablePort
  VIPR4sStEnCtrl_Cal : FunctionCaller  FunctionPrototype=VIPR4sStEnCtrl_Cal()

== system ModeStEnCtrl4s/ModeStEnCtrl4s_Cal_sys/Subsystem/EZEStEnCtrl3 ==
  note: Delete block
  Enable : EnablePort
  RecvR4sStEnCtrl_Cal : FunctionCaller  FunctionPrototype=RecvR4sStEnCtrl_Cal()

== system ModeStEnCtrl4s/ModeStEnCtrl4s_Cal_sys/Subsystem/EZEStEnCtrl4 ==
  note: Delete block
  Enable : EnablePort
  LyRStEnCtrl_Cal : FunctionCaller  FunctionPrototype=LyRStEnCtrl_Cal()

== system ModeStEnCtrl4s/ModeStEnCtrl4s_Cal_sys/Subsystem/EZEStEnCtrl5 ==
  note: Delete block
  Enable : EnablePort
  LyLStEnCtrl_Cal : FunctionCaller  FunctionPrototype=LyLStEnCtrl_Cal()

== system ModeStEnCtrl4s/ModeStEnCtrl4s_Cal_sys/Subsystem/EZEStEnCtrl6 ==
  note: Delete block
  Enable : EnablePort
  LgrstOpnLStEnCtrl_Cal : FunctionCaller  FunctionPrototype=LgrstOpnLStEnCtrl_Cal()

== system ModeStEnCtrl4s/ModeStEnCtrl4s_Cal_sys/Subsystem/EZEStEnCtrl7 ==
  note: Delete block
  Enable : EnablePort
  LgrstClsLStEnCtrl_Cal : FunctionCaller  FunctionPrototype=LgrstClsLStEnCtrl_Cal()

== system ModeStEnCtrl4s/ModeStEnCtrl4s_Cal_sys/Subsystem/EZEStEnCtrl8 ==
  note: Delete block
  Enable : EnablePort
  LgrstOpnRStEnCtrl_Cal : FunctionCaller  FunctionPrototype=LgrstOpnRStEnCtrl_Cal()

== system ModeStEnCtrl4s/ModeStEnCtrl4s_Cal_sys/Subsystem/EZEStEnCtrl9 ==
  note: Delete block
  Enable : EnablePort
  LgrstClsRStEnCtrl_Cal : FunctionCaller  FunctionPrototype=LgrstClsRStEnCtrl_Cal()
